simulink model "c2812iqsinetest"  (Simulink 6.0)
settings: Solver=FixedStepDiscrete  StartTime=0.0  StopTime=2  RelTol=1e-3
StopFcn:
  | runc2812iqsine('Simulation')
libraries: tiiqmathlib x15, memblks x3, c2000tgtpreflib x1
settings Model: Creator=maydinli  LastModifiedBy=mkachmar  ProdHWDeviceType=TI C2000
settings DataIOCC: SignalLoggingName=sigsOut
settings OptimizationCC: InlineInvariantSignals=off  EnforceIntegerDowncast=off  ExpressionFolding=off  FoldNonRolledExpr=off  LocalBlockOutputs=off
settings DebuggingCC: CheckExecutionContextPreStartOutputMsg=on  CheckExecutionContextRuntimeOutputMsg=on  SolverPrmCheckMsg=none
settings HardwareCC: ProdBitPerChar=16  ProdBitPerInt=16  ProdIntDivRoundTo=Zero  ProdEndianess=LittleEndian  ProdWordSize=16  ProdHWDeviceType=TI C2000
settings ModelReferenceCC: UpdateModelReferenceTargets=IfOutOfDate
settings RTWCC: SystemTargetFile=ti_c2000_grt.tlc  GenCodeOnly=on  TemplateMakefile=ti_c2000_grt.tmf  ProcessScript=ti_c2000_grt_make_rtw_hook
settings STFCustomTargetCC: TargetFcnLib=ansi_tfl_tmw.mat  GenFloatMathFcnCalls=ANSI_C  ModelReferenceCompliant=off  SystemTargetFile=ti_c2000_grt.tlc  ActivateCallback=ti_c2000_callback('ActivateCallback',hSrc,hDlg);  ForcedBaseTarget=off
settings GRTTargetCC: ModelReferenceCompliant=off  MatFileLogging=off
settings SFSimCC: SFSimApplyToAllLibs=on  SFSimBuildMode=Incremental

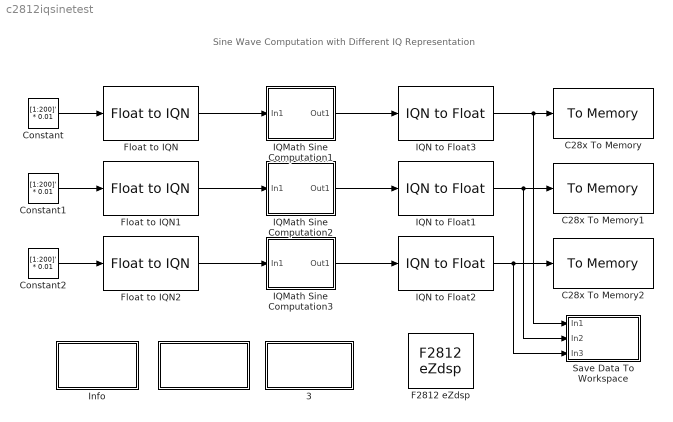
== system c2812iqsinetest ==
  note: Sine Wave Computation with Different IQ Representation
  " " : Subsystem  PropExecContextAcrossSSBoundary=on
      settings: OpenFcn=runc2812iqsine('Build_Run')
      mask Type: Run demo
      mask Display: disp(sprintf('Build & Run'))
  " 3" : Subsystem  PropExecContextAcrossSSBoundary=on
      settings: OpenFcn=runc2812iqsine('Reload_Run')
      mask Type: Run demo
      mask Display: disp(sprintf('Reload & Run'))
  " Info" : Subsystem  PropExecContextAcrossSSBoundary=on
      mask Display: disp('Info')
  C28x To Memory : memblks/To Memory  memAddressMask=8000  dType=single  useInitValue=on  initValue=0  useTermValue=off  termValue=0  isRealtimeEnabled=on
  C28x To Memory1 : memblks/To Memory  memAddressMask=8320  dType=single  useInitValue=on  initValue=0  useTermValue=off  termValue=0  isRealtimeEnabled=on
  C28x To Memory2 : memblks/To Memory  memAddressMask=8640  dType=single  useInitValue=on  initValue=0  useTermValue=off  termValue=0  isRealtimeEnabled=on
  Constant : Constant  Value=[1:200]' * 0.01  VectorParams1D=off  OutDataTypeMode=single  SampleTime=0.1
  Constant1 : Constant  Value=[1:200]' * 0.01  VectorParams1D=off  OutDataTypeMode=single  SampleTime=0.1
  Constant2 : Constant  Value=[1:200]' * 0.01  VectorParams1D=off  OutDataTypeMode=single  SampleTime=0.1
  F2812 eZdsp : c2000tgtpreflib/F2812 eZdsp  Tag=C2000 TARGET PREFERENCES BLOCK
  Float to IQN : tiiqmathlib/Float to IQN  Q_value=4
  Float to IQN1 : tiiqmathlib/Float to IQN  Q_value=5
  Float to IQN2 : tiiqmathlib/Float to IQN  Q_value=15
  IQMath Sine Computation1 : Subsystem  PropExecContextAcrossSSBoundary=on
  IQMath Sine Computation2 : Subsystem  PropExecContextAcrossSSBoundary=on
  IQMath Sine Computation3 : Subsystem  PropExecContextAcrossSSBoundary=on
  IQN to Float1 : tiiqmathlib/IQN to Float
  IQN to Float2 : tiiqmathlib/IQN to Float
  IQN to Float3 : tiiqmathlib/IQN to Float
  Save Data To Workspace : Subsystem  PropExecContextAcrossSSBoundary=on
  wires:
  Constant/1 -> Float to IQN/1
  Float to IQN/1 -> IQMath Sine Computation1/1(In1)
  IQMath Sine Computation1/1(Out1) -> IQN to Float3/1
  IQN to Float3/1 -> C28x To Memory/1, Save Data To Workspace/1(In1)
  Constant1/1 -> Float to IQN1/1
  Float to IQN1/1 -> IQMath Sine Computation2/1(In1)
  IQMath Sine Computation2/1(Out1) -> IQN to Float1/1
  Constant2/1 -> Float to IQN2/1
  Float to IQN2/1 -> IQMath Sine Computation3/1(In1)
  IQMath Sine Computation3/1(Out1) -> IQN to Float2/1
  IQN to Float2/1 -> C28x To Memory2/1, Save Data To Workspace/3(In3)
  IQN to Float1/1 -> C28x To Memory1/1, Save Data To Workspace/2(In2)

== system c2812iqsinetest/  ==

== system c2812iqsinetest/ 3 ==

== system c2812iqsinetest/ Info ==
  note: This example demonstrates how to use the IQ math library blocks that come with
      | the embedded Target for TIC2000 product. These blocks support simulation and
      | code generation. This simple demo computes the fixed point sine result of
      | floating-point input values using different IQN representations, and plots it.
      |
      | The "Float to IQN" blocks convert the floating-point input values to fixed-point using
      | the equivalent Q-value parameter in the block. The sine computation is also
      | done using IQ math blocks in fixed-point, and then the values are converted to
      | floating-point again using the "IQN to Float block".
  note: Demo Description:
  note: Run the Demo:
  note: To run the demo, you can simply simulate , or double click on the "Build & Run"
      | button to generate code and run on the target. "Reload & Run" will load the existing
      | COFF file and run it again.

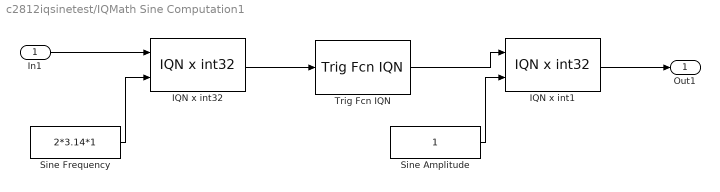
== system c2812iqsinetest/IQMath Sine Computation1 ==
  In1 : Inport  LatchInput=off
  IQN x int1 : tiiqmathlib/IQN x int32
  IQN x int32 : tiiqmathlib/IQN x int32
  Sine Amplitude : Constant  VectorParams1D=off  OutDataTypeMode=int32  SampleTime=0.1
  Sine Frequency : Constant  Value=2*3.14*1  VectorParams1D=off  OutDataTypeMode=int32  SampleTime=0.1
  Trig Fcn IQN : tiiqmathlib/Trig Fcn IQN  functionOption=_IQsin
  Out1 : Outport
  wires:
  Sine Frequency/1 -> IQN x int32/2
  Sine Amplitude/1 -> IQN x int1/2
  IQN x int1/1 -> Out1/1
  In1/1 -> IQN x int32/1
  IQN x int32/1 -> Trig Fcn IQN/1
  Trig Fcn IQN/1 -> IQN x int1/1

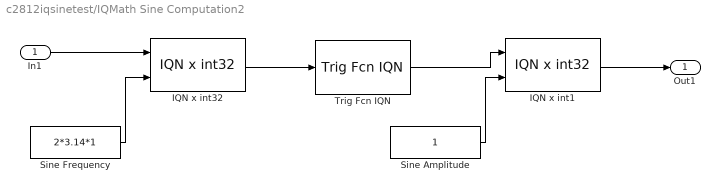
== system c2812iqsinetest/IQMath Sine Computation2 ==
  In1 : Inport  LatchInput=off
  IQN x int1 : tiiqmathlib/IQN x int32
  IQN x int32 : tiiqmathlib/IQN x int32
  Sine Amplitude : Constant  VectorParams1D=off  OutDataTypeMode=int32  SampleTime=0.1
  Sine Frequency : Constant  Value=2*3.14*1  VectorParams1D=off  OutDataTypeMode=int32  SampleTime=0.1
  Trig Fcn IQN : tiiqmathlib/Trig Fcn IQN  functionOption=_IQsin
  Out1 : Outport
  wires:
  Trig Fcn IQN/1 -> IQN x int1/1
  IQN x int32/1 -> Trig Fcn IQN/1
  In1/1 -> IQN x int32/1
  IQN x int1/1 -> Out1/1
  Sine Amplitude/1 -> IQN x int1/2
  Sine Frequency/1 -> IQN x int32/2

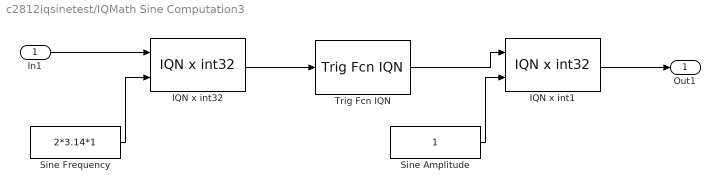
== system c2812iqsinetest/IQMath Sine Computation3 ==
  In1 : Inport  LatchInput=off
  IQN x int1 : tiiqmathlib/IQN x int32
  IQN x int32 : tiiqmathlib/IQN x int32
  Sine Amplitude : Constant  VectorParams1D=off  OutDataTypeMode=int32  SampleTime=0.1
  Sine Frequency : Constant  Value=2*3.14*1  VectorParams1D=off  OutDataTypeMode=int32  SampleTime=0.1
  Trig Fcn IQN : tiiqmathlib/Trig Fcn IQN  functionOption=_IQsin
  Out1 : Outport
  wires:
  Sine Frequency/1 -> IQN x int32/2
  Sine Amplitude/1 -> IQN x int1/2
  IQN x int1/1 -> Out1/1
  In1/1 -> IQN x int32/1
  IQN x int32/1 -> Trig Fcn IQN/1
  Trig Fcn IQN/1 -> IQN x int1/1

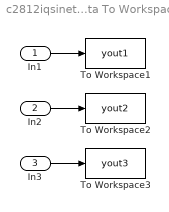
== system c2812iqsinetest/Save Data To Workspace ==
  In1 : Inport  LatchInput=off
  In2 : Inport  Port=2  LatchInput=off
  In3 : Inport  Port=3  LatchInput=off
  To Workspace1 : ToWorkspace  VariableName=yout1  SampleTime=-1  SaveFormat=Structure
      settings: MaxDataPoints=200
  To Workspace2 : ToWorkspace  VariableName=yout2  SampleTime=-1  SaveFormat=Structure
  To Workspace3 : ToWorkspace  VariableName=yout3  SampleTime=-1  SaveFormat=Structure
  wires:
  In1/1 -> To Workspace1/1
  In2/1 -> To Workspace2/1
  In3/1 -> To Workspace3/1
